simulink model "ClosedLoop"  (R2018b)
settings: Solver=FixedStepAuto  StartTime=0.0  StopTime=10.0  FixedStep=0.02  RelTol=1e-3
libraries: neural x506, simulink x1
(part 12 of 12)

== system ClosedLoop/Controller/Layer 3/Delays 1 ==
  "p{3}" : Inport  PortDimensions=200
      mask Display: e = 0.06;c1 = [120 230 180]/255;c2 = ([120 230 180]+0)/(256+128);c3 = ([120 230 180]+128)/(256+128);patch([0 1 1 0],[0 0 1 1],c1);patch([0 1 1 1-e 1-e 0+e],[0 0 1 1-e 0+e 0+e],c2);patch([0 0 1 1-e 0+e 0+e],[0 1 1 1-e 1-e 0+e],c3);plot([0 1 1 0 0],[0 0 1 1 0]);
  mux : Mux  Inputs=1
      mask Display: e = 0.06;c1 = [120 150 230]/255;c2 = ([120 150 230]+0)/383;c3 = ([120 150 230]+128)/383;patch([0 1 1 0],[0 0 1 1],c1);patch([0 1 1 1-e 1-e 0+e],[0 0 1 1-e 0+e 0+e],c2);patch([0 0 1 1-e 0+e 0+e],[0 1 1 1-e 1-e 0+e],c3);plot([0 1 1 0 0],[0 0 1 1 0]);disp('Mux')
  "pd{3,2}" : Outport
      mask Display: e = 0.06;c1 = [120 230 180]/255;c2 = ([120 230 180]+0)/(256+128);c3 = ([120 230 180]+128)/(256+128);patch([0 1 1 0],[0 0 1 1],c1);patch([0 1 1 1-e 1-e 0+e],[0 0 1 1-e 0+e 0+e],c2);patch([0 0 1 1-e 0+e 0+e],[0 1 1 1-e 1-e 0+e],c3);plot([0 1 1 0 0],[0 0 1 1 0]);
  wires:
  mux/1 -> "pd{3,2}"/1
  "p{3}"/1 -> mux/1

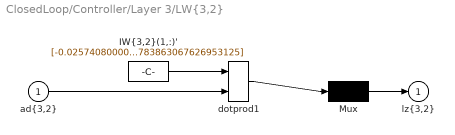
== system ClosedLoop/Controller/Layer 3/LW{3,2} ==
  "ad{3,2}" : Inport  PortDimensions=200
      mask Display: e = 0.06;c1 = [120 230 180]/255;c2 = ([120 230 180]+0)/(256+128);c3 = ([120 230 180]+128)/(256+128);patch([0 1 1 0],[0 0 1 1],c1);patch([0 1 1 1-e 1-e 0+e],[0 0 1 1-e 0+e 0+e],c2);patch([0 0 1 1-e 0+e 0+e],[0 1 1 1-e 1-e 0+e],c3);plot([0 1 1 0 0],[0 0 1 1 0]);
  "IW{3,2}(1,:)'" : Constant  Value=[-0.025740800000000001179767394887676346115767955780029296875;0.10361800000000000177013959046234958805143833160400390625;-0.12257099999999999939692685302361496724188327789306640625;0.018558999999999999108712955830924329347908496856689453125;-0.0372335000000000027053914664065814577043056488037109375;0.00436578999999999960157648359881932265125215053558349609375;-0.1257810000000000039133141171987517736852169036865234375;-0.025193000000000000115907283770866342820227146148681640625;-0.0088840599999999991798205201121163554489612579345703125;-0.00964418000000000046056936042759843985550105571746826171875;0.00672034999999999993480770399401080794632434844970703125;-0.021939199999999998980104720658346195705235004425048828125;-0.01224699999999999920630155969547558925114572048187255859375;-0.0915616999999999958692598056586575694382190704345703125;0.0446734000000000019969803588537615723907947540283203125;0.01962529999999999830162522584942053072154521942138671875;-0.01053270000000000074236172764585717231966555118560791015625;-0.0017148400000000000274746891903987489058636128902435302734375;-0.0063987200000000001021138729129233979620039463043212890625;-0.0201169999999999994655386359454496414400637149810791015625;-0.07759810000000000318465254167676903307437896728515625;-0.0062812600000000003153122207777414587326347827911376953125;0.0502907999999999966167507636782829649746417999267578125;-0.05413500000000000256239474083486129529774188995361328125;-0.019508299999999999252420224138404591940343379974365234375;-0.011553000000000000768718422250458388589322566986083984375;0.0144496999999999993502530770683733862824738025665283203125;0.01028970000000000058204552288998456788249313831329345703125;-0.0196150999999999998968380765518304542638361454010009765625;0.02096610000000000140207845333861769177019596099853515625;-0.136747000000000007435829729729448445141315460205078125;-0.0028536299999999997951960484243727478315122425556182861328125;0.0037559099999999998910349408021147610270418226718902587890625;-0.00108146999999999995738242386522642846102826297283172607421875;0.010797199999999999853184107223569299094378948211669921875;0.38451000000000001843858399297459982335567474365234375;0.00572890000000000031155078517031142837367951869964599609375;0.06535059999999999480468915180608746595680713653564453125;-0.1490579999999999960547114596920437179505825042724609375;-0.08961529999999999496207436777694965712726116180419921875;-0.0303380000000000003834710327055290690623223781585693359375;-0.043488199999999997691357833673464483581483364105224609375;0.00938934999999999943265382995605250471271574497222900390625;-0.047089600000000002288924605409192736260592937469482421875;-0.06530850000000000543654010698446654714643955230712890625;-0.02398139999999999993907096040857140906155109405517578125;-0.0021694499999999998507416165693939547054469585418701171875;-0.0264260000000000015718537582642966299317777156829833984375;-0.028663399999999998601918349550032871775329113006591796875;-0.1009420000000000039452885403079562820494174957275390625;-0.028415900000000000880095996080854092724621295928955078125;-0.0013815599999999999929201077719653767417185008525848388671875;-0.07153410000000000323883142527847667224705219268798828125;-0.09572029999999999427817698460785322822630405426025390625;0.0004071599999999999980500320351239906813134439289569854736328125;0.0029159899999999998147781621327112588915042579174041748046875;-0.0127057999999999997331467938010973739437758922576904296875;0.0191056999999999997663646666978820576332509517669677734375;-0.018166700000000000903010999309117323718965053558349609375;-0.0209756000000000004945821530100147356279194355010986328125;-0.14941199999999998926369926266488619148731231689453125;0.387056000000000011151968237754772417247295379638671875;0.003291230000000000023574475704890573979355394840240478515625;-0.0186364000000000008816503083153293118812143802642822265625;-0.09053129999999999510951198544717044569551944732666015625 ...(+8174 chars)]
      mask Display: e = 0.06;c1 = [120 150 230]/255;c2 = ([120 150 230]+0)/383;c3 = ([120 150 230]+128)/383;patch([0 1 1 0],[0 0 1 1],c1);patch([0 1 1 1-e 1-e 0+e],[0 0 1 1-e 0+e 0+e],c2);patch([0 0 1 1-e 0+e 0+e],[0 1 1 1-e 1-e 0+e],c3);plot([0 1 1 0 0],[0 0 1 1 0]);disp('weights');
  Mux : Mux  Inputs=1
      mask Display: e = 0.06;c1 = [120 150 230]/255;c2 = ([120 150 230]+0)/383;c3 = ([120 150 230]+128)/383;patch([0 1 1 0],[0 0 1 1],c1);patch([0 1 1 1-e 1-e 0+e],[0 0 1 1-e 0+e 0+e],c2);patch([0 0 1 1-e 0+e 0+e],[0 1 1 1-e 1-e 0+e],c3);plot([0 1 1 0 0],[0 0 1 1 0]);disp('Mux');
  dotprod1 : neural/Weight Functions/dotprod
  "lz{3,2}" : Outport
      mask Display: e = 0.06;c1 = [120 230 180]/255;c2 = ([120 230 180]+0)/(256+128);c3 = ([120 230 180]+128)/(256+128);patch([0 1 1 0],[0 0 1 1],c1);patch([0 1 1 1-e 1-e 0+e],[0 0 1 1-e 0+e 0+e],c2);patch([0 0 1 1-e 0+e 0+e],[0 1 1 1-e 1-e 0+e],c3);plot([0 1 1 0 0],[0 0 1 1 0]);
  wires:
  Mux/1 -> "lz{3,2}"/1
  dotprod1/1 -> Mux/1
  "ad{3,2}"/1 -> dotprod1/2
  "IW{3,2}(1,:)'"/1 -> dotprod1/1

== system ClosedLoop/Controller/Layer 4/Delays 1 ==
  "p{4}" : Inport  PortDimensions=1
      mask Display: e = 0.06;c1 = [120 230 180]/255;c2 = ([120 230 180]+0)/(256+128);c3 = ([120 230 180]+128)/(256+128);patch([0 1 1 0],[0 0 1 1],c1);patch([0 1 1 1-e 1-e 0+e],[0 0 1 1-e 0+e 0+e],c2);patch([0 0 1 1-e 0+e 0+e],[0 1 1 1-e 1-e 0+e],c3);plot([0 1 1 0 0],[0 0 1 1 0]);
  mux : Mux  Inputs=1
      mask Display: e = 0.06;c1 = [120 150 230]/255;c2 = ([120 150 230]+0)/383;c3 = ([120 150 230]+128)/383;patch([0 1 1 0],[0 0 1 1],c1);patch([0 1 1 1-e 1-e 0+e],[0 0 1 1-e 0+e 0+e],c2);patch([0 0 1 1-e 0+e 0+e],[0 1 1 1-e 1-e 0+e],c3);plot([0 1 1 0 0],[0 0 1 1 0]);disp('Mux')
  "pd{4,3}" : Outport
      mask Display: e = 0.06;c1 = [120 230 180]/255;c2 = ([120 230 180]+0)/(256+128);c3 = ([120 230 180]+128)/(256+128);patch([0 1 1 0],[0 0 1 1],c1);patch([0 1 1 1-e 1-e 0+e],[0 0 1 1-e 0+e 0+e],c2);patch([0 0 1 1-e 0+e 0+e],[0 1 1 1-e 1-e 0+e],c3);plot([0 1 1 0 0],[0 0 1 1 0]);
  wires:
  mux/1 -> "pd{4,3}"/1
  "p{4}"/1 -> mux/1

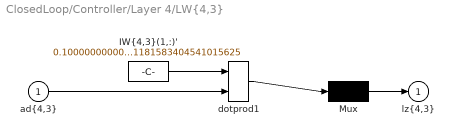
== system ClosedLoop/Controller/Layer 4/LW{4,3} ==
  "ad{4,3}" : Inport  PortDimensions=1
      mask Display: e = 0.06;c1 = [120 230 180]/255;c2 = ([120 230 180]+0)/(256+128);c3 = ([120 230 180]+128)/(256+128);patch([0 1 1 0],[0 0 1 1],c1);patch([0 1 1 1-e 1-e 0+e],[0 0 1 1-e 0+e 0+e],c2);patch([0 0 1 1-e 0+e 0+e],[0 1 1 1-e 1-e 0+e],c3);plot([0 1 1 0 0],[0 0 1 1 0]);
  "IW{4,3}(1,:)'" : Constant  Value=0.1000000000000000055511151231257827021181583404541015625
      mask Display: e = 0.06;c1 = [120 150 230]/255;c2 = ([120 150 230]+0)/383;c3 = ([120 150 230]+128)/383;patch([0 1 1 0],[0 0 1 1],c1);patch([0 1 1 1-e 1-e 0+e],[0 0 1 1-e 0+e 0+e],c2);patch([0 0 1 1-e 0+e 0+e],[0 1 1 1-e 1-e 0+e],c3);plot([0 1 1 0 0],[0 0 1 1 0]);disp('weights');
  Mux : Mux  Inputs=1
      mask Display: e = 0.06;c1 = [120 150 230]/255;c2 = ([120 150 230]+0)/383;c3 = ([120 150 230]+128)/383;patch([0 1 1 0],[0 0 1 1],c1);patch([0 1 1 1-e 1-e 0+e],[0 0 1 1-e 0+e 0+e],c2);patch([0 0 1 1-e 0+e 0+e],[0 1 1 1-e 1-e 0+e],c3);plot([0 1 1 0 0],[0 0 1 1 0]);disp('Mux');
  dotprod1 : neural/Weight Functions/dotprod
  "lz{4,3}" : Outport
      mask Display: e = 0.06;c1 = [120 230 180]/255;c2 = ([120 230 180]+0)/(256+128);c3 = ([120 230 180]+128)/(256+128);patch([0 1 1 0],[0 0 1 1],c1);patch([0 1 1 1-e 1-e 0+e],[0 0 1 1-e 0+e 0+e],c2);patch([0 0 1 1-e 0+e 0+e],[0 1 1 1-e 1-e 0+e],c3);plot([0 1 1 0 0],[0 0 1 1 0]);
  wires:
  Mux/1 -> "lz{4,3}"/1
  dotprod1/1 -> Mux/1
  "ad{4,3}"/1 -> dotprod1/2
  "IW{4,3}(1,:)'"/1 -> dotprod1/1

== stateflow chart ClosedLoop/Plant ==
  settings: updateMethod=CONTINUOUS
  state b1
    du:
    x1_dot = x3^3 - x2 + w;
    x2_dot = x3;
    x3_dot = u;
    % Outputs
    x1_out = x1;
    x2_out = x2;
    x3_out = x3;
  (default) -> b1 : {x1 = 0.4;
      | x2 = 0.5;
      | x3 = 0.3}
  data: u input; w input; x1_out output; x2_out output; x1 local; x2 local; x3 local; x3_out output
  data x1 settings: updateMethod=SF_CONTINUOUS_TIME_DATA
  data x2 settings: updateMethod=SF_CONTINUOUS_TIME_DATA
  data x3 settings: updateMethod=SF_CONTINUOUS_TIME_DATA
